simulink model "qcm_baseband"  (R2026a)
settings: Solver=VariableStepAuto  StopTime=2
model workspace (MAT data in the model file):
  Framesize = 1000
  Fs = 100000
libraries: dspsrcs4 x2, commchan3 x1, commrflib2 x1
settings Model: Creator=ranja  LastModifiedBy=ranja

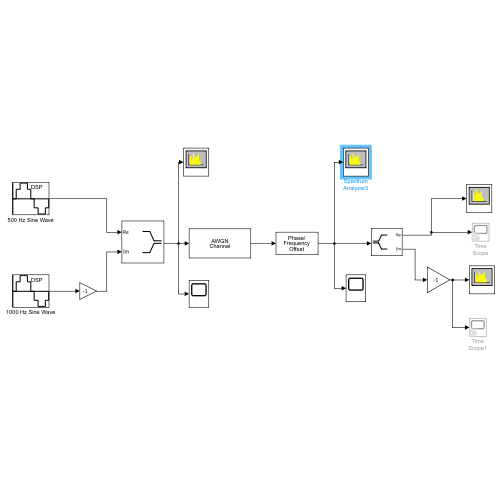
[thumbnail: Simulink's stored preview of the top-level diagram]
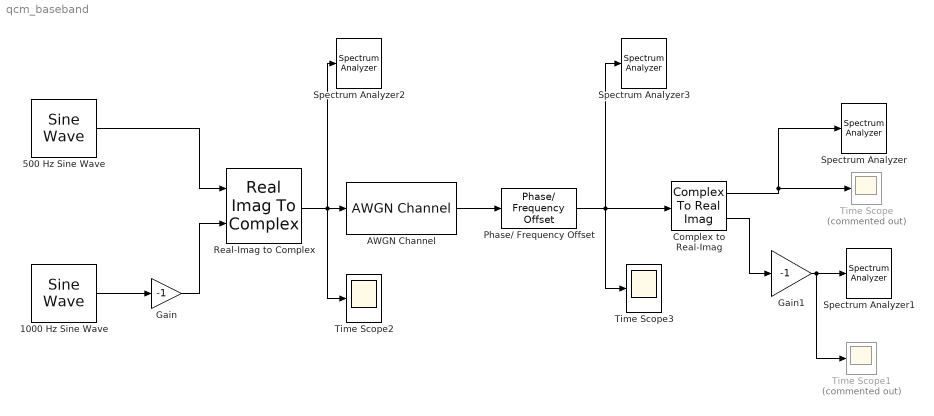
== system qcm_baseband ==
  1000 Hz Sine Wave : dspsrcs4/Sine Wave  Amplitude=1  Frequency=1000  Phase=0  SampleMode=Discrete  OutComplex=Real  CompMethod=Trigonometric fcn  TableSize=Speed  SampleTime=1/Fs  SamplesPerFrame=Framesize  ResetState=Restart at time zero  OutputFrames=off  dataType=double  wordLen=16  udDataType=sfix(16)  fracBitsMode=Best precision  numFracBits=15  OutDataTypeStr=double  LastOutDataTypeStr=double
  500 Hz Sine Wave : dspsrcs4/Sine Wave  Amplitude=1  Frequency=500  Phase=0  SampleMode=Discrete  OutComplex=Real  CompMethod=Trigonometric fcn  TableSize=Speed  SampleTime=1/Fs  SamplesPerFrame=Framesize  ResetState=Restart at time zero  OutputFrames=off  dataType=double  wordLen=16  udDataType=sfix(16)  fracBitsMode=Best precision  numFracBits=15  OutDataTypeStr=double  LastOutDataTypeStr=double
  AWGN Channel : commchan3/AWGN Channel  LegacyMode=off  NoiseMethod="Signal to noise ratio  (SNR)"  noiseMode="Signal to noise ratio  (SNR)"  EbNo=10  EsNo=10  SNR=20  BitsPerSymbol=1  SignalPower=1  SpecifySymbolPeriod=off  SamplesPerSymbol=1  SymbolPeriod=1  VarianceSource=Parameter  Variance=1  RandomStream=Global stream  Seed=67  SimulateUsing=Code generation
  Complex to Real-Imag : ComplexToRealImag
  Gain : Gain  Gain=-1
  Gain1 : Gain  Gain=-1
  Phase/ Frequency Offset : commrflib2/Phase// Frequency Offset  PhaseOffset=30  FrequencyOffsetFromPort=off  FrequencyOffset=50  SimulateUsing=Code generation
  Real-Imag to Complex : RealImagToComplex
  Spectrum Analyzer : SpectrumAnalyzer  WindowPosition=[1.000000,49.000000,1536.000000,793.000000,]  ScopeFrameLocation=window  WindowInvariantSamplesPerUpdate=on  FrequencySpan=Span and center frequency  Span=5000  YLimits=[-65.7446 11.1878]  SelectedToolstripTab=spectrumAnalyzerToolstrip.estimationTab
  Spectrum Analyzer1 : SpectrumAnalyzer  WindowPosition=[387.000000,-12.000000,800.000000,500.000000,]  ScopeFrameLocation=window  WindowInvariantSamplesPerUpdate=on  FrequencySpan=Span and center frequency  Span=5000  YLimits=[-58.2664 10.1976]  SelectedToolstripTab=spectrumAnalyzerToolstrip.spectrumTab
  Spectrum Analyzer2 : SpectrumAnalyzer  WindowPosition=[368.000000,182.000000,800.000000,500.000000,]  ScopeFrameLocation=window  WindowInvariantSamplesPerUpdate=on  FrequencySpan=Span and center frequency  Span=5000  YLimits=[-143.37000863374394 47.35208895082575]  SelectedToolstripTab=spectrumAnalyzerToolstrip.estimationTab
  Spectrum Analyzer3 : SpectrumAnalyzer  WindowPosition=[1.000000,49.000000,1536.000000,793.000000,]  ScopeFrameLocation=window  WindowInvariantSamplesPerUpdate=on  FrequencySpan=Span and center frequency  Span=5000  YLimits=[-76.0136353094241 19.762381394534565]  SelectedToolstripTab=spectrumAnalyzerToolstrip.estimationTab
  Time Scope : Scope  Commented=on
      settings: TimeUnits=Metric (based on Time Span)  ActiveDisplayYMinimum=-1.864704003098657  ActiveDisplayYMaximum=1.8572987573008495  YLabel=Amplitude
  Time Scope1 : Scope  Commented=on
      settings: TimeUnits=Metric (based on Time Span)  ActiveDisplayYMinimum=-1.8403783197481447  ActiveDisplayYMaximum=1.8392110805668596  YLabel=Amplitude
  Time Scope2 : Scope
      settings: TimeUnits=Metric (based on Time Span)  ActiveDisplayYMinimum=-1.2880090083479336  ActiveDisplayYMaximum=1.1766332764775735  YLabel=Amplitude  DataLoggingVariableName=ScopeData2
  Time Scope3 : Scope
      settings: TimeUnits=Metric (based on Time Span)  YLabel=Amplitude  DataLoggingVariableName=ScopeData3
  wires:
  1000 Hz Sine Wave/1 -> Gain/1
  500 Hz Sine Wave/1 -> Real-Imag to Complex/1
  Gain/1 -> Real-Imag to Complex/2
  Real-Imag to Complex/1 -> Time Scope2/1, Spectrum Analyzer2/1, AWGN Channel/1
  AWGN Channel/1 -> Phase/ Frequency Offset/1
  Complex to Real-Imag/2 -> Gain1/1
  Complex to Real-Imag/1 -> Spectrum Analyzer/1, Time Scope/1
  Gain1/1 -> Time Scope1/1, Spectrum Analyzer1/1
  Phase/ Frequency Offset/1 -> Time Scope3/1, Spectrum Analyzer3/1, Complex to Real-Imag/1
